simulink model "Fzgsym_MtrSpd"  (R2022a)
settings: Solver=VariableStepAuto  StartTime=0.0  StopTime=100  RelTol=1e-3
values from neighbouring files (symbols this model uses):
  g = 9.81    [Energiebedarf_single.m]
  m = 1500    [Energiebedarf_single.m]
undefined symbols (not defined in the file or in its folder): air_temp, battPwrChrgLmt, battPwrDischrgLmt, brkprs_front, brkprs_max, brkprs_rear, disk_abore, efficiency, l_CG_rear, mass_veh, mu_kinetic, nmo_rpm, num_mot, num_pads, r_m, trq, trq_eff
libraries: simulink x8, autolibshared x7, autolibmappedmotor x4, autolibutils x1, autolibdatasheetbattery x1
(part 1 of 4)
settings Model: Creator=ferdi  LastModifiedBy=ferdi

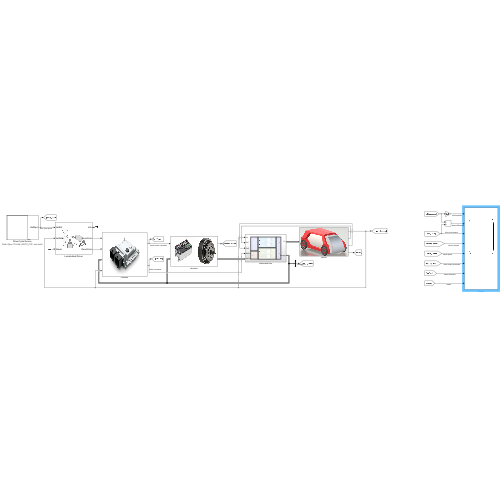
[thumbnail: Simulink's stored preview of the top-level diagram]
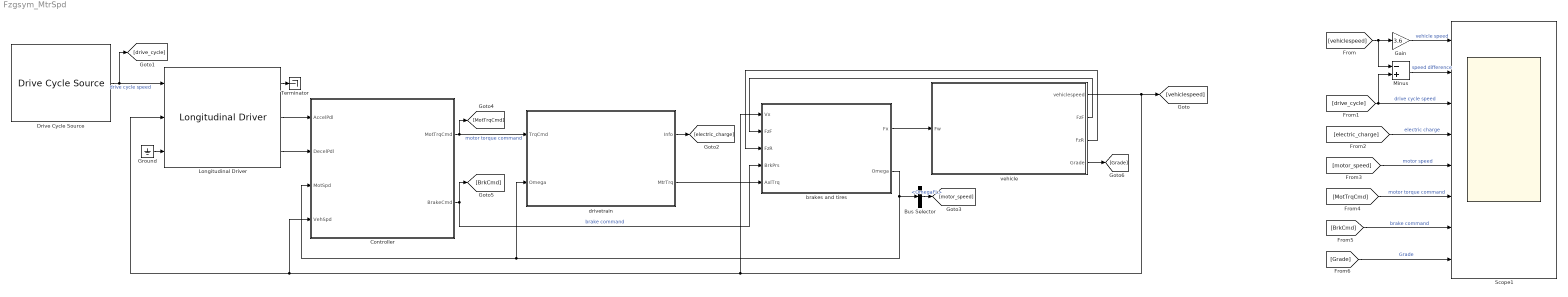
== system Fzgsym_MtrSpd ==
  Bus Selector : BusSelector  OutputSignals=OmegaFL
  Controller : Subsystem
      mask Display: image('ECU'); % Use "Edit Image" on toolstrip to change.
  Drive Cycle Source : autolibshared/Drive Cycle Source  cycleVar=Wide Open Throttle (WOT)  fileVar=C:\Users\ferdi\OneDrive\Dokumente\MATLAB\Hiwi\HElmar\WLTC.mat  tfinal="100  seconds"  cycleRepeat=off  outAccPort=off  outGearPort=off  gearList=No gear data  t_wot1=2  xdot_woto=0  xdot_wot1=50  t_wot2=90  xdot_wot2=0  t_wotend=100  srcUnit=m/s  outUnit=m/s  srcAccUnit=m/s/s  outAccUnit=m/s^2  dt=0  aMode=1  faultOption=off  velBnd=2  velBndUnit=mph  inUnit=m/s  timeBnd=1  failOption=off  stopSim=off  maxFaultCnt=10  maxFaultTime=2  maxTotFaultTime=15  traceOption=off  dtTrace=1  traceWindow=10  lastDCname=Custom Data Set  lastOutUnit=mph  lastDT=0  lastTB=1  lastSB=2  forceCalcBound=off
      settings: SourceProductBaseCode=PW,DR,MT,VE
  Gain : Gain  Gain=3.6
  Ground : Ground
  Longitudinal Driver : autolibshared/Longitudinal Driver  extAccelOvr=off  extDecelOvr=off  extAccelHld=off  extDecelHld=off  extAccelZero=off  extDecelZero=off  cntrlType=PI  shftType=None  velUnits=m/s  gearOut=off  Kp=5  Ki=25  Kff=.05  Kg=0.01  VehVelVec=gain_velocity  KffVec=gain_velocity_ff  KpVec=gain_proportional  KiVec=gain_integral  KgVec=grade_angle_ff  m=780  Kpt=3000  tau=.1  L=10  aR=200  bR=2.5  cR=.5  g=9.81  vnom=v_nom  Kaw=kaw  tauerr=tauerr  tauPt=2  GearInit=0  tShift=.1  pdlVec=[0.1 0.4 0.5 0.9]  upShftTbl=[-1 12.9375 26.4375 39.9375 51.18749999999999 62.4375 72.84375 83.25;-1 16.3125 29.8125 43.3125 54.5624 65.8125 76.78125 87.75;-1 19.6875 33.1875 46.68749999999999 57.9375 69.1875 80.71875 92.25;-1 33 52.5 77.25 100.5 138.75 161.875 185]  dwnShftTbl=[1 9.5625 23.0625 36.5625 47.8125 59.0625 68.90625 78.75;1 12.9375 26.4375 39.9375 51.18749999999999 62.4375 72.84375 83.25;1 16.3125 29.8125 43.3125 54.562499 65.8125 76.78125 87.75;1 19.6875 33.1875 46.68749999999999 57.9375 69.1875 80.71875 92.25]  tClutch=.5  tRev=.5  tPark=120  aMode=1  UpGearVec="[0  1  2  3  4  5  6  7]"  DownGearVec="[1  2  3  4  5  6  7  8]"
      settings: SourceProductBaseCode=PW,DR,MT,VE
  Minus : Sum  Inputs=-+
  Scope1 : Scope  NumInputPorts=8
  Terminator : Terminator
  brakes and tires : Subsystem
  drivetrain : Subsystem
      mask Display: image('Batterie_Motor.png'); % Use "Edit Image" on toolstrip to change.
  vehicle : Subsystem
      mask Display: image('HEImar.png'); % Use "Edit Image" on toolstrip to change.
  wires:
  Drive Cycle Source/1 -> Longitudinal Driver/1, [drive_cycle]  "drive cycle speed"
  Ground/1 -> Longitudinal Driver/3
  Longitudinal Driver/2 -> Controller/1(AccelPdl)
  Longitudinal Driver/3 -> Controller/2(DecelPdl)
  brakes and tires/2(Omega) -> Bus Selector/1, drivetrain/2(Omega), Controller/3(MotSpd)
  Controller/2(BrakeCmd) -> brakes and tires/4(BrkPrs), [BrkCmd]  "brake command"
  vehicle/1(vehiclespeed) -> Longitudinal Driver/2, Controller/4(VehSpd), brakes and tires/1(Vx), [vehiclespeed]
  vehicle/2(FzF) -> brakes and tires/2(FzF)
  vehicle/3(FzR) -> brakes and tires/3(FzR)
  Controller/1(MotTrqCmd) -> [MotTrqCmd], drivetrain/1(TrqCmd)  "motor torque command"
  Longitudinal Driver/1 -> Terminator/1
  brakes and tires/1(Fx) -> vehicle/1(Fw)
  drivetrain/2(MtrTrq) -> brakes and tires/5(AxlTrq)
  [vehiclespeed] -> Minus/1, Gain/1
  [drive_cycle] -> Minus/2, Scope1/3  "drive cycle speed"
  drivetrain/1(Info) -> [electric_charge]
  [electric_charge] -> Scope1/4  "electric charge"
  Bus Selector/1 -> [motor_speed]  "<OmegaFL>"
  [motor_speed] -> Scope1/5  "motor speed"
  [BrkCmd] -> Scope1/7  "brake command"
  [MotTrqCmd] -> Scope1/6  "motor torque command"
  Gain/1 -> Scope1/1  "vehicle speed"
  Minus/1 -> Scope1/2  "speed difference"
  vehicle/4(Grade) -> [Grade]
  [Grade] -> Scope1/8  "Grade"

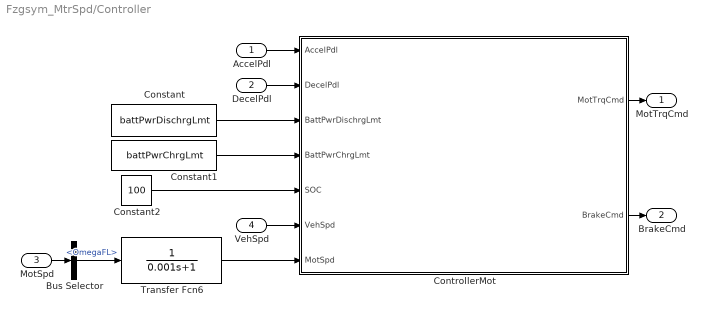
== system Fzgsym_MtrSpd/Controller ==
  AccelPdl : Inport
  DecelPdl : Inport  Port=2
  MotSpd : Inport  Port=3
  VehSpd : Inport  Port=4
  Bus Selector : BusSelector  OutputSignals=OmegaFL
  Constant : Constant  Value=battPwrDischrgLmt
  Constant1 : Constant  Value=battPwrChrgLmt
  Constant2 : Constant  Value=100
  ControllerMot : Subsystem
  Transfer Fcn6 : TransferFcn  Denominator=[0.001 1]
  MotTrqCmd : Outport
  BrakeCmd : Outport  Port=2
  wires:
  AccelPdl/1 -> ControllerMot/1(AccelPdl)
  VehSpd/1 -> ControllerMot/6(VehSpd)
  DecelPdl/1 -> ControllerMot/2(DecelPdl)
  ControllerMot/1(MotTrqCmd) -> MotTrqCmd/1
  ControllerMot/2(BrakeCmd) -> BrakeCmd/1
  Constant2/1 -> ControllerMot/5(SOC)
  Constant1/1 -> ControllerMot/4(BattPwrChrgLmt)
  Constant/1 -> ControllerMot/3(BattPwrDischrgLmt)
  MotSpd/1 -> Bus Selector/1
  Bus Selector/1 -> Transfer Fcn6/1  "<OmegaFL>"
  Transfer Fcn6/1 -> ControllerMot/7(MotSpd)
